simulink model "scenario_II"  (R2025a)
settings: Solver=VariableStepAuto  StartTime=0.0  StopTime=5  RelTol=1e-3
undefined symbols (not defined in the file): C, L, R, Ts_Power
libraries: spsSeriesRLCBranchLib x4, powerlib_extras x2, spsVoltageMeasurementLib x2, spsCurrentMeasurementLib x2, spsDiodeLib x1, spsIGBTLib x1, spsPWMGeneratorDCDCLib x1, spsControlledVoltageSourceLib x1, spsDCVoltageSourceLib x1, spspowerguiLib x1
settings Model: SimulationMode=accelerator  Creator=User  LastModifiedBy=md-saiful-islam
settings DebuggingCC: UnconnectedInputMsg=warning  UnconnectedOutputMsg=warning  UnconnectedLineMsg=warning
settings ModelReferenceCC: EnableRefExpFcnMdlSchedulingChecks=on
settings RTWCC: GPUComputeCapability=3.5  DLArmComputeVersion=19.05

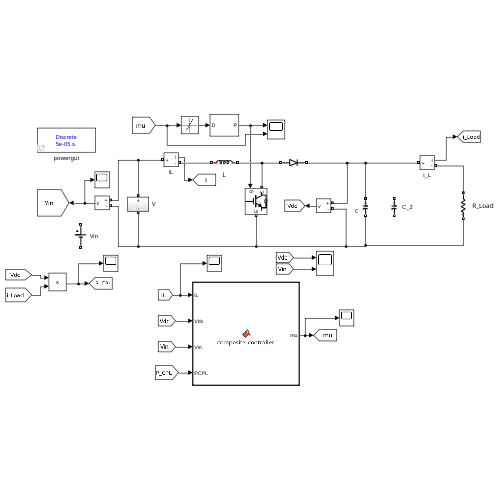
[thumbnail: Simulink's stored preview of the top-level diagram]
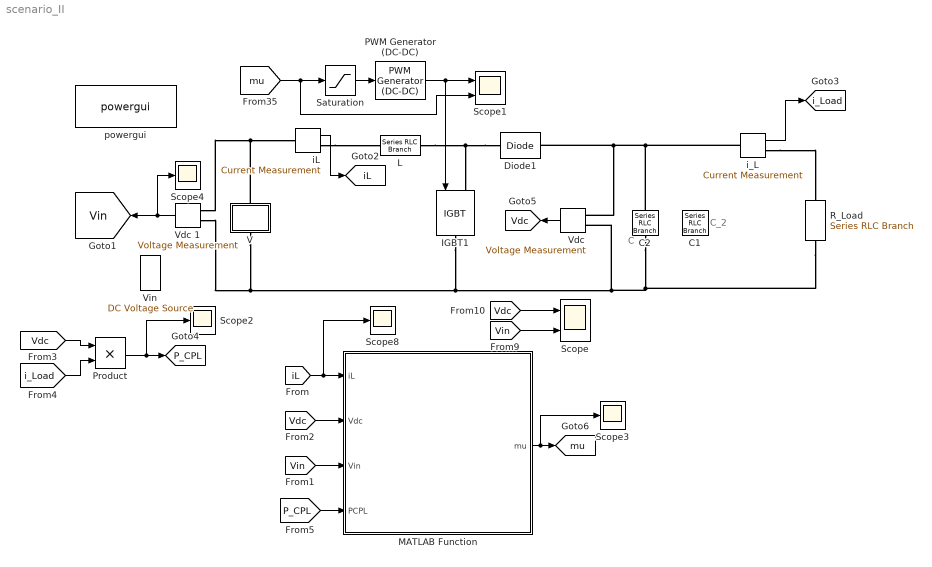
== system scenario_II ==
  note: C
  note: C_2
  C1 : spsSeriesRLCBranchLib/Series RLC Branch  LConnTagsString=__new0  RConnTagsString=__new0  BranchType=C  Resistance=1.0  Inductance=1.0  SetiL0=off  InitialCurrent=0  Capacitance=10*C  Setx0=off  InitialVoltage=0  Measurements=None
  C2 : spsSeriesRLCBranchLib/Series RLC Branch  LConnTagsString=__new0  RConnTagsString=__new0  BranchType=C  Resistance=1.0  Inductance=1.0  SetiL0=off  InitialCurrent=0  Capacitance=0.0060933  Setx0=off  InitialVoltage=0  Measurements=None
  Diode1 : spsDiodeLib/Diode  Ron=1e-4  Lon=0  Vf=0  IC=0  UseSnubber=off  Rs=inf  Cs=inf  Measurements=off
  IGBT1 : spsIGBTLib/IGBT  Ron=0.0001  Lon=0  Vf=0  Tf=0  Tt=0  IC=0  Rs=1e5  Cs=inf  Measurements=off
  L : spsSeriesRLCBranchLib/Series RLC Branch  LConnTagsString=__new0  RConnTagsString=__new0  BranchType=L  Resistance=R  Inductance=0.0105  SetiL0=off  InitialCurrent=0  Capacitance=1e-6  Setx0=off  InitialVoltage=0  Measurements=None
  MATLAB Function : MATLAB Function  TreatAsAtomicUnit=on
  PWM Generator (DC-DC) : spsPWMGeneratorDCDCLib/PWM Generator (DC-DC)  Fsw=fc  Ts=1e-4
  Product : Product  OutDataTypeStr=Inherit: Keep MSB
  R_Load : spsSeriesRLCBranchLib/Series RLC Branch  LConnTagsString=__new0  RConnTagsString=__new0  BranchType=R  Resistance=4.1263  Inductance=L  SetiL0=off  InitialCurrent=0  Capacitance=1e-6  Setx0=off  InitialVoltage=0  Measurements=None
  Saturation : Saturate  UpperLimit=1  LowerLimit=0
  Scope : Scope  NumInputPorts=2
      settings: ShowGrid=off  ActiveDisplayYMinimum=-14.6499  ActiveDisplayYMaximum=131.85399
  Scope1 : Scope  NumInputPorts=2
      settings: ActiveDisplayYMinimum=-0.41394  ActiveDisplayYMaximum=1.49255  DataLoggingVariableName=ScopeData2
  Scope{2..4,8} (4 alike) : Scope
      Scope2 settings: ShowGrid=off  ActiveDisplayYMinimum=-462.81404  ActiveDisplayYMaximum=4165.32638
      Scope3 settings: ShowGrid=off  ActiveDisplayYMinimum=-2.72946  ActiveDisplayYMaximum=1.24058  DataLoggingVariableName=ScopeData3
      Scope4 settings: ShowGrid=off  ActiveDisplayYMinimum=38.75  ActiveDisplayYMaximum=51.25  DataLoggingVariableName=ScopeData4
      Scope8 settings: ShowGrid=off  ActiveDisplayYMinimum=-9.80463  ActiveDisplayYMaximum=89.43418  DataLoggingVariableName=ScopeData8
  V : Subsystem
  "Vdc " : spsVoltageMeasurementLib/Voltage Measurement  Tag=PoWeRsYsTeMmEaSuReMeNt  PhasorSimulation=off  OutputType=Magnitude  PSBequivalent=0
  Vdc 1 : spsVoltageMeasurementLib/Voltage Measurement  Tag=PoWeRsYsTeMmEaSuReMeNt  PhasorSimulation=off  OutputType=Magnitude  PSBequivalent=0
  Vin : spsDCVoltageSourceLib/DC Voltage Source  Amplitude=50  Measurements=None
  iL : spsCurrentMeasurementLib/Current Measurement  PhasorSimulation=off  OutputType=Complex  PSBequivalent=0
  i_L : spsCurrentMeasurementLib/Current Measurement  PhasorSimulation=off  OutputType=Complex  PSBequivalent=0
  powergui : spspowerguiLib/powergui  Priority=1  SimulationMode=Discrete  SampleTime=Ts_Power  frequency=60  Iterations=50  frequencyindice=0  Pbase=100e6  ErrMax=1e-4  UnitsV=kV  UnitsW=MW  buscounter=0  FunctionMessages=off  echomessages=off  EnableUseOfTLC=off  CurrentSourceSwitches=off  DisableSnubberDevices=off  DisableRonSwitches=off  DisableVfSwitches=off  DisplayEquations=off  AutomaticDiscreteSolvers=off  SolverType=Tustin/Backward Euler (TBE)  Interpol=off  ExternalGateDelay=off  methode=off  Ts=100  x0status=blocks  SPID=on  SwTol=0  HookPort=off  NonlinearTolerance=1e-4  nMaxIteration=100  ContinueOnMaxIteration=off  RestoreLinks=warning  ResistiveCurrentMeasurement=off  Frange=[0:2:500]  Ylog=off  Xlog=on  ShowGrid=off  save=off  variable=ZData  structure=0  ZoomFFT=on  StartTime=0.0  cycles=1  DisplayStyle=1  fundamental=60  FreqAxis=off  MaxFrequency=1000  frequencyindicesteady=1  RmsSteady=1  display=off
  tag scope: P_CPL=global, Vdc=global, Vin=global, iL=global, i_Load=global, mu=global
  wires:
  "Vdc "/1 -> [Vdc]
  Vdc 1/1 -> Scope4/1, [Vin]
  [mu] -> Scope1/2, Saturation/1
  iL/1 -> [iL]
  Saturation/1 -> PWM Generator (DC-DC)/1
  i_L/1 -> [i_Load]
  PWM Generator (DC-DC)/1 -> Scope1/1, IGBT1/1
  [iL] -> Scope8/1, MATLAB Function/1(iL)
  [Vin] -> MATLAB Function/3(Vin)
  [Vdc] -> MATLAB Function/2(Vdc)
  [Vdc] -> Product/1
  [i_Load] -> Product/2
  Product/1 -> Scope2/1, [P_CPL]
  [P_CPL] -> MATLAB Function/4(PCPL)
  MATLAB Function/1(mu) -> Scope3/1, [mu]
  [Vdc] -> Scope/1
  [Vin] -> Scope/2
  connections:
  Vdc 1/LConn1 -- V/RConn1 -- iL/LConn1
  IGBT1/RConn1 -- V/LConn1 -- Vdc 1/LConn2 -- R_Load/LConn1 -- C2/RConn1 -- "Vdc "/LConn2
  "Vdc "/LConn1 -- i_L/LConn1 -- C2/LConn1 -- Diode1/RConn1
  Diode1/LConn1 -- IGBT1/LConn1 -- L/RConn1
  i_L/RConn1 -- R_Load/RConn1
  iL/RConn1 -- L/LConn1

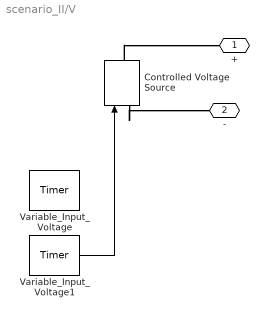
== system scenario_II/V ==
  Controlled Voltage Source : spsControlledVoltageSourceLib/Controlled Voltage Source  Initialize=on  Source_Type=AC  Amplitude=0  Phase=0  Frequency=0  Measurements=None
  Variable_Input_Voltage : powerlib_extras/Control  Blocks/Timer  t=[0, 0.7, 0.8]  e=[50, 40, 50]
  Variable_Input_Voltage1 : powerlib_extras/Control  Blocks/Timer  t=[0, 0.7, 0.8, 1.4, 1.5, 3.5, 3.6, 4.4, 4.5]  e=[50, 40, 50, 40, 50, 40, 50, 40, 50]
  + : PMIOPort  Side=Right
  - : PMIOPort  Port=2  Side=Left
  wires:
  Variable_Input_Voltage1/1 -> Controlled Voltage Source/1
  connections:
  Controlled Voltage Source/RConn1 -- +/RConn1
  Controlled Voltage Source/LConn1 -- -/RConn1

== matlab function scenario_II/MATLAB Function ==
  data: iL input; mu output; Vdc input; Vin input; PCPL input
function mu = composite_controller(iL, Vdc, Vin, PCPL)

%% system parameters
R     = 5.1579;    
L     = 0.0105;    
Cdc   = 5.5394e-04;  
Cvir  = 5.5394e-04;  
C  = Cdc + Cvir;

%% Reference values
Vdc_ref     = 100;            

% Controller parameters
K1   = 2000;
K2   = 50;
K3   = 5;
Kub1 = 1;
Kub2 = 1;

% Sliding surface and IFPRL params
a_surf = 0.2;
b_surf = 0.1;
num    = 3;
den    = 5;
p      = 0.6;

% Sample time
Ts = 1e-4;

%% -------- persistent states --------
persistent I_e2 m1_prev Vdc_prev init Vint
if isempty(init)
    I_e2     = 0.0;  % ∫ e2 dt
    m1_prev  = 0.0;  % prev m1
    Vdc_prev = 0.0;  % prev Vdc
    Vint     = 0.0;  % integral for voltage loop
    init     = true;
end

%% -------- small safeties --------
eps_b   = 1e-6;
eps_pow = 1e-9;
eps_sgn = 1e-12;

%% -------- voltage regulation--------
eV = Vdc_ref - Vdc;        % voltage error
Kp_v = 60;                % proportional gain Kp_v = 0.5
Ki_v = 400;                % integral gain Ki_v = 200
Vint = Vint + Ts*eV;       % integral
Vc_ref = Kp_v*eV + Ki_v*Vint;  % virtual reference for inductor current

%% -------- compute m1, m2 --------
m1 = 0.5*L*iL^2 + 0.5*C*Vdc^2;
if m1_prev == 0
    m2 = 0.0;
else
    m2 = (m1 - m1_prev)/Ts;
end
m1_prev = m1;

%% -------- Vdc derivative for ΔPvir --------
if Vdc_prev == 0
    dVdc = 0.0;
else
    dVdc = (Vdc - Vdc_prev)/Ts;
end
Vdc_prev = Vdc;
DeltaPvir = Vdc * Cvir * dVdc;

%% -------- errors & virtual control Λ --------
iL_ref = Vc_ref / max(Vin,1e-3);  % avoid divide by zero
m1_ref      = 0.5*L*iL_ref^2 + 0.5*C*Vdc_ref^2;
m1_ref_dot  = 0.0;            
m1_ref_ddot = 0.0;

e1 = m1 - m1_ref;
Lambda = -K1*e1 + m1_ref_dot;
e2 = m2 - Lambda;

%% -------- accumulate ∫e2 --------
I_e2 = I_e2 + Ts*e2;

%% -------- fractional power for sliding surface --------
pow_int_e2 = sign_preserving_pow(I_e2, num/den, eps_pow);
alpha = num/den;
pow_int_e2_minus1 = sign(I_e2) * (abs(I_e2) + eps_pow)^(alpha - 1);

%% -------- sliding surface S --------
S = e2 + a_surf*I_e2 + b_surf*pow_int_e2;
if abs(S) < eps_sgn
    sgnS = 0.0;
else
    sgnS = sign(S);
end

%% -------- a(x) and b(x) --------
a_x = (Vin*(Vin - Vdc))/L ...
      - (2*Vdc)/(R*C) * ( iL - Vdc/R + (DeltaPvir)/Vdc - (PCPL)/Vdc );

b_x = (Vin*Vdc)/L + (2*iL*Vdc)/(R*C);
if abs(b_x) < eps_b
    b_safe = sign(b_x + (b_x==0)) * eps_b;
else
    b_safe = b_x;
end

%% -------- tau --------
tau = -K1*(m2 - m1_ref_dot) + m1_ref_ddot;

%% -------- control law --------
term_lin_int = a_surf*e2;
term_frac    = (b_surf*(num/den)) * e2 * pow_int_e2_minus1;

reach_const  = (K2 + Kub1 + Kub2) * sgnS;
reach_frac   = K3 * (abs(S))^p * sgnS;

mu = -(1.0 / b_safe) * ( a_x - tau + term_lin_int + term_frac + reach_const + reach_frac );

%% -------- saturate duty cycle --------
mu = max(0, min(1, mu));  % ensure mu ∈ [0,1]

%% -------- helper function --------
    function y = sign_preserving_pow(z, alpha, epsv)
        if z > 0
            y = z^alpha;
        elseif z < 0
            y = -((-z)^alpha);
        else
            y = 0.0;
        end
        if abs(z) < epsv
            y = 0.0;
        end
    end

end
